simulink subsystem "Calculate_FF"  (R2022b)
settings: Solver=VariableStepAuto  StartTime=0.0  StopTime=10.0  RelTol=1e-3
libraries: matrix_library x1
settings Model: Creator=hollis  LastModifiedBy=hollis

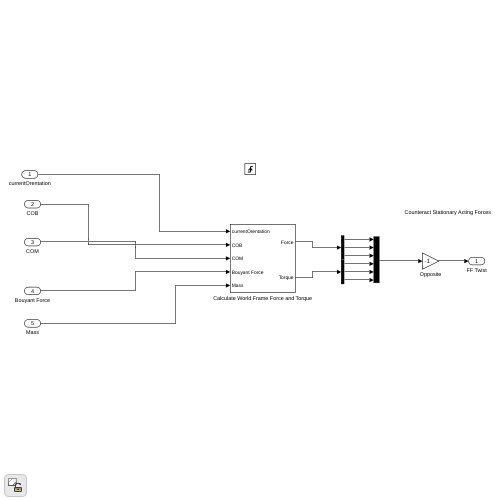
[thumbnail: Simulink's stored preview of the top-level diagram]
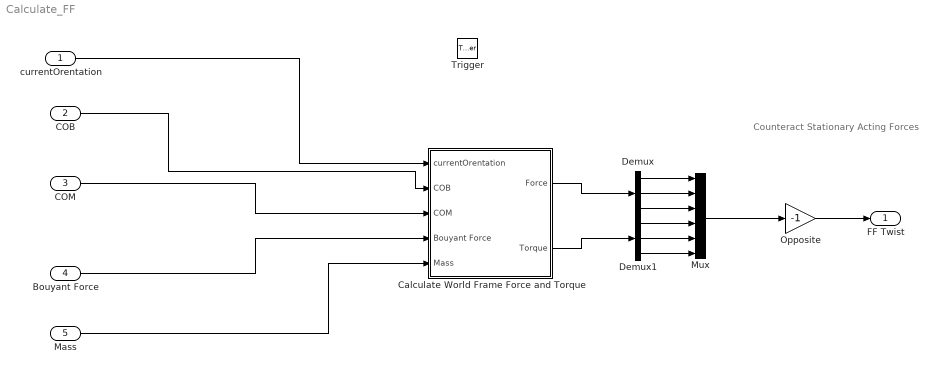
== system Calculate_FF ==
  note: Counteract Stationary Acting Forces
  currentOrentation : Inport
  COB : Inport  Port=2
  COM : Inport  Port=3
  Bouyant Force : Inport  Port=4
  Mass : Inport  Port=5
  Trigger : TriggerPort  VariantControl=(inherit)  PortDimensions=1
  Calculate World Frame Force and Torque : Subsystem
  Demux : Demux  Outputs=3
  Demux1 : Demux  Outputs=3
  Mux : Mux  Inputs=6
  Opposite : Gain  Gain=-1
  FF Twist : Outport
  wires:
  Calculate World Frame Force and Torque/1(Force) -> Demux/1
  Opposite/1 -> FF Twist/1
  currentOrentation/1 -> Calculate World Frame Force and Torque/1(currentOrentation)
  Demux1/2 -> Mux/5
  COM/1 -> Calculate World Frame Force and Torque/3(COM)
  Demux/2 -> Mux/2
  Mux/1 -> Opposite/1
  Calculate World Frame Force and Torque/2(Torque) -> Demux1/1
  COB/1 -> Calculate World Frame Force and Torque/2(COB)
  Demux/1 -> Mux/1
  Demux1/3 -> Mux/6
  Demux1/1 -> Mux/4
  Demux/3 -> Mux/3
  Mass/1 -> Calculate World Frame Force and Torque/5(Mass)
  Bouyant Force/1 -> Calculate World Frame Force and Torque/4(Bouyant Force)

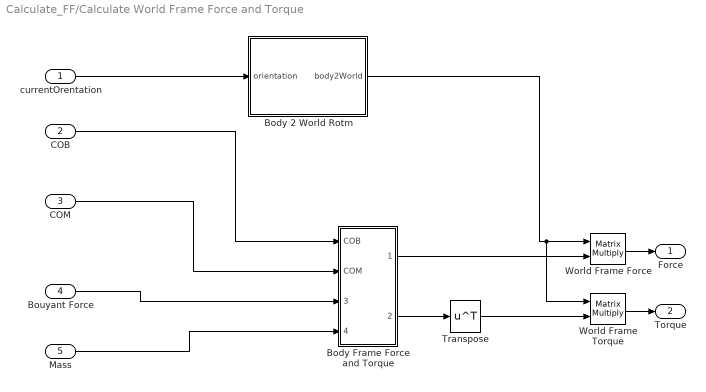
== system Calculate_FF/Calculate World Frame Force and Torque ==
  currentOrentation : Inport
  COB : Inport  Port=2
  COM : Inport  Port=3
  Bouyant Force : Inport  Port=4
  Mass : Inport  Port=5
  Body 2 World Rotm : MATLAB Function  TreatAsAtomicUnit=on
  Body Frame Force and Torque : Subsystem
  Transpose : Math  Operator=transpose
  World Frame Force : Product  Multiplication=Matrix(*)
  World Frame Torque : Product  Multiplication=Matrix(*)
  Force : Outport
  Torque : Outport  Port=2
  wires:
  Transpose/1 -> World Frame Torque/2
  currentOrentation/1 -> Body 2 World Rotm/1(orientation)
  Body 2 World Rotm/1(body2World) -> World Frame Force/1, World Frame Torque/1
  World Frame Force/1 -> Force/1
  Body Frame Force and Torque/2(torque) -> Transpose/1
  Body Frame Force and Torque/1(force) -> World Frame Force/2
  World Frame Torque/1 -> Torque/1
  Mass/1 -> Body Frame Force and Torque/4(Mass)
  COB/1 -> Body Frame Force and Torque/1(COB)
  COM/1 -> Body Frame Force and Torque/2(COM)
  Bouyant Force/1 -> Body Frame Force and Torque/3(Bouyant Force)

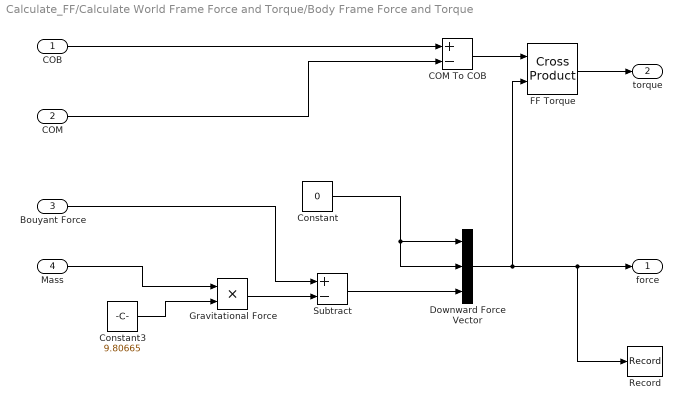
== system Calculate_FF/Calculate World Frame Force and Torque/Body Frame Force and Torque ==
  COB : Inport
  COM : Inport  Port=2
  Bouyant Force : Inport  Port=3
  Mass : Inport  Port=4
  COM To COB : Sum  Inputs=+-
  Constant : Constant  Value=0
  Constant3 : Constant  Value=9.80665
  Downward Force Vector : Mux  Inputs=3
  FF Torque : matrix_library/Cross Product
  Gravitational Force : Product
  Record : Record  FileSettingsInternal="{\"entries\":[{\"content\":{\"excelSettings\":{\"content\":{},\"type\":\"Streamout.ExcelSettings\"}},\"type\":\"Streamout.FileSettingStorage\",\"uuid\":\"3f97c42d-4bed-4617-88e2-ac8d6fbf9365\"}],\"packageUris\":[\"http://schema.mathworks.com/mf0/streamout_blocks/R2020a\"],\"version\":\"1.0\"}"  SignalsInternal="{\"entries\":[{\"content\":{\"signals\":[]},\"type\":\"RecordBlkView.InputSignals\",\"uuid\":\"7a778385-6bb3-4161-bab8-825a86ceece4\"}],\"packageUris\":[\"http://schema.mathworks.com/mf0/streamout_blocks/R2020a\"],\"version\":\"1.0\"}"  VisualizationBindings="{\"sparklinesplugin\":{\"info\":[{\"bindingParametersList\":[],\"subplotID\":1}]}}"
  Subtract : Sum  Inputs=+-
  force : Outport
  torque : Outport  Port=2
  wires:
  Bouyant Force/1 -> Subtract/1
  Mass/1 -> Gravitational Force/1
  Constant3/1 -> Gravitational Force/2
  COB/1 -> COM To COB/1
  FF Torque/1 -> torque/1
  COM/1 -> COM To COB/2
  Gravitational Force/1 -> Subtract/2
  Subtract/1 -> Downward Force Vector/3
  Downward Force Vector/1 -> FF Torque/2, force/1, Record/1
  Constant/1 -> Downward Force Vector/2, Downward Force Vector/1
  COM To COB/1 -> FF Torque/1

== matlab function Calculate_FF/Calculate World Frame Force and Torque/Body 2 World Rotm ==
  data: orientation input; body2World output
function body2World = fcn(orientation)

%ros2 quaternion order to matlab quaternion order
quaternion = [orientation(4), orientation(1), orientation(2), orientation(3)];

%world to body frame rotation
world2body = quat2rotm(quaternion);

%transpose rotm = inverse
body2World = transpose(world2body);
